simulink model "problem3"  (R2020b)
settings: Solver=ode45  StartTime=0.0  StopTime=120  RelTol=1e-3
model workspace (MAT data in the model file):
  Ki = Simulink.Parameter
  Ki.Value = 40
  Ki.DataType = 'auto'
  Ki.Dimensions = [1 1]
  Kp = Simulink.Parameter
  Kp.Value = 800
  Kp.DataType = 'auto'
  Kp.Dimensions = [1 1]
  b = Simulink.Parameter
  b.Value = 50
  b.DataType = 'auto'
  b.Dimensions = [1 1]
  m = Simulink.Parameter
  m.Value = 1000
  m.DataType = 'auto'
  m.Dimensions = [1 1]
  u = Simulink.Parameter
  u.Value = 500
  u.DataType = 'auto'
  u.Dimensions = [1 1]
settings Model: Creator=admin  LastModifiedBy=admin

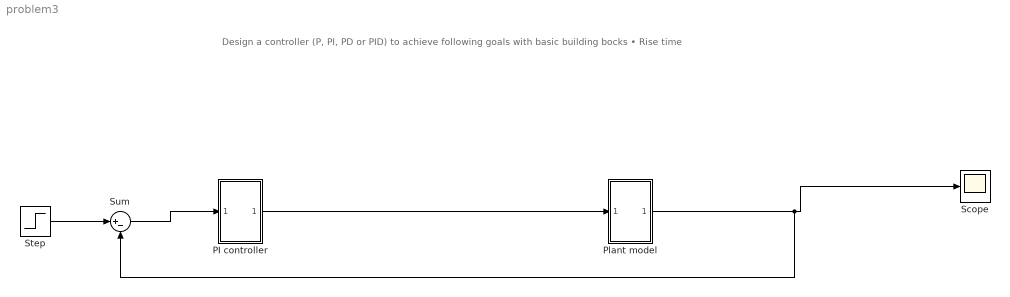
== system problem3 ==
  note: Design a controller (P, PI, PD or PID) to achieve following goals with basic building bocks • Rise time
  PI controller : Subsystem
  Plant model : Subsystem
  Scope : Scope
  Step : Step  SampleTime=0
  Sum : Sum  Inputs=|+-
  wires:
  Plant model/1(Out1) -> Scope/1, Sum/2
  PI controller/1(Out2) -> Plant model/1(In1)
  Step/1 -> Sum/1
  Sum/1 -> PI controller/1(In2)

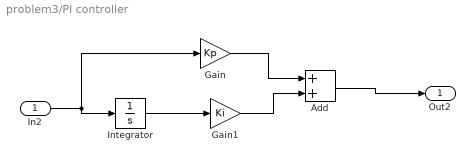
== system problem3/PI controller ==
  In2 : Inport
  Add : Sum
  Gain : Gain  Gain=Kp
  Gain1 : Gain  Gain=Ki
  Integrator : Integrator
  Out2 : Outport
  wires:
  Gain1/1 -> Add/2
  Add/1 -> Out2/1
  Integrator/1 -> Gain1/1
  In2/1 -> Integrator/1, Gain/1
  Gain/1 -> Add/1

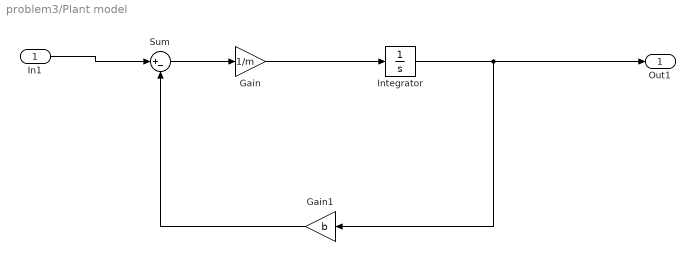
== system problem3/Plant model ==
  In1 : Inport
  Gain : Gain  Gain=1/m
  Gain1 : Gain  Gain=b
  Integrator : Integrator
  Sum : Sum  Inputs=|+-
  Out1 : Outport
  wires:
  Sum/1 -> Gain/1
  In1/1 -> Sum/1
  Gain1/1 -> Sum/2
  Gain/1 -> Integrator/1
  Integrator/1 -> Out1/1, Gain1/1
